simulink model "lptmr_complex_time_counter_s32k11x"  (Simulink 9.0)
settings: Solver=FixedStepDiscrete  StartTime=0.0  StopTime=10.0  FixedStep=0.1  RelTol=1e-3
InitFcn:
  | mbd_s32k_consistency_checks(bdroot(gcs));
undefined symbols (not defined in the file): LQFP, thumb
libraries: mbd_s32k1xx_ec_toolbox x12, simulink x1
Description:
  | This model demonstrates the "Low Power Timer" functionality by setting the peripheral to work in Time counter mode and using most of the LPTMR blocks.
  | 
  | Validation: When the processor boots up, it configures the LPTMR timer to Time Counter mode at an initial time period  of 1 sec and also enables the ISR. At every LPTMR
  |  interrup callback the model gets the compare value and toggles it between 50 or 950 msecs, so the RGB led will lightd up 50 msecs green at every second. On every step
  | function, the model gets the counter value and compares it to 55k Ticks and and the RGB led will lights up red if the counter value is higher than 50k Ticks. The counter can
  | be stopped if the SW3 switch is pressed and can be started if the SW2 switch is pressed.
settings Model: Creator=NXP MBDT Team  LastModifiedBy=nxf35172
settings DataIOCC: ExternalInput=off  InitialState=off  SaveFormat=Dataset  SaveOutput=off  SignalLogging=off  SaveTime=off
settings OptimizationCC: DefaultParameterBehavior=Inlined  PassReuseOutputArgsAs=Individual arguments  LifeSpan=auto
settings DebuggingCC: UnderspecifiedInitializationDetection=Simplified  MergeDetectMultiDrivingBlocksExec=error  InheritedTsInSrcMsg=none  SingleTaskRateTransMsg=error  ParameterTunabilityLossMsg=error  UnconnectedInputMsg=error  UnconnectedOutputMsg=error  UnconnectedLineMsg=error  UnknownTsInhSupMsg=error  SFUnexpectedBacktrackingDiag=error  SFNoUnconditionalDefaultTransitionDiag=error  SFExecutionAtInitializationDiag=warning
settings HardwareCC: ProdLargestAtomicInteger=Long  ProdLargestAtomicFloat=Double  ProdIntDivRoundTo=Zero  ProdEndianess=LittleEndian  ProdHWDeviceType=ARM Compatible->ARM Cortex
settings ModelReferenceCC: PropagateSignalLabelsOutOfModel=on
settings SFSimCC: MATLABDynamicMemAlloc=off
settings RTWCC: SystemTargetFile=mbd_s32k.tlc  MakeCommand=mbd_s32k_make_rtw COPY_MDLREF_INCLUDES=0  TemplateMakefile=mbd_s32k.tmf  Description=Model Based Design Toolbox S32K14x Code Generation Target  GenerateReport=on  IncludeHyperlinkInReport=on  LaunchReport=on  GenerateTraceInfo=on  GenerateTraceReport=on  GenerateTraceReportSl=on  GenerateTraceReportSf=on  GenerateTraceReportEml=on
settings CodeAppCC: ForceParamTrailComments=on  IgnoreCustomStorageClasses=off  OperatorAnnotations=on  SimulinkDataObjDesc=on  SFDataObjDesc=on  InsertBlockDesc=on  StateflowObjectComments=off
settings STFCustomTargetCC: TargetLangStandard=C99 (ISO)  MultiwordLength=256  CombineOutputUpdateFcns=on  ERTCustomFileBanners=on  SupportContinuousTime=off  SupportNonInlinedSFcns=off  RemoveResetFunc=on  MATLABClassNameForMDSCustomization=Simulink.SoftwareTarget.ERTCustomization  GRTInterface=off  SystemTargetFile=mbd_s32k.tlc
settings ERTTargetCC: TargetLangStandard=C99 (ISO)  ParMdlRefBuildCompliant=off  CompOptLevelCompliant=off  ConcurrentExecutionCompliant=off  ModelStepFunctionPrototypeControlCompliant=off  CPPClassGenCompliant=off  UseToolchainInfoCompliant=off  InlinedParameterPlacement=NonHierarchical  ERTSrcFileBannerTemplate=mbd_ert_code_template.cgt  ERTHdrFileBannerTemplate=mbd_ert_code_template.cgt  ERTDataSrcFileTemplate=mbd_ert_code_template.cgt  ERTDataHdrFileTemplate=mbd_ert_code_template.cgt  ERTCustomFileTemplate=example_file_process.tlc
settings ConfigComp: CovMetricSettings=dwe  CovHtmlReporting=off  CovSaveCumulativeToWorkspaceVar=off  CovSaveSingleToWorkspaceVar=off  CovExternalEMLEnable=on

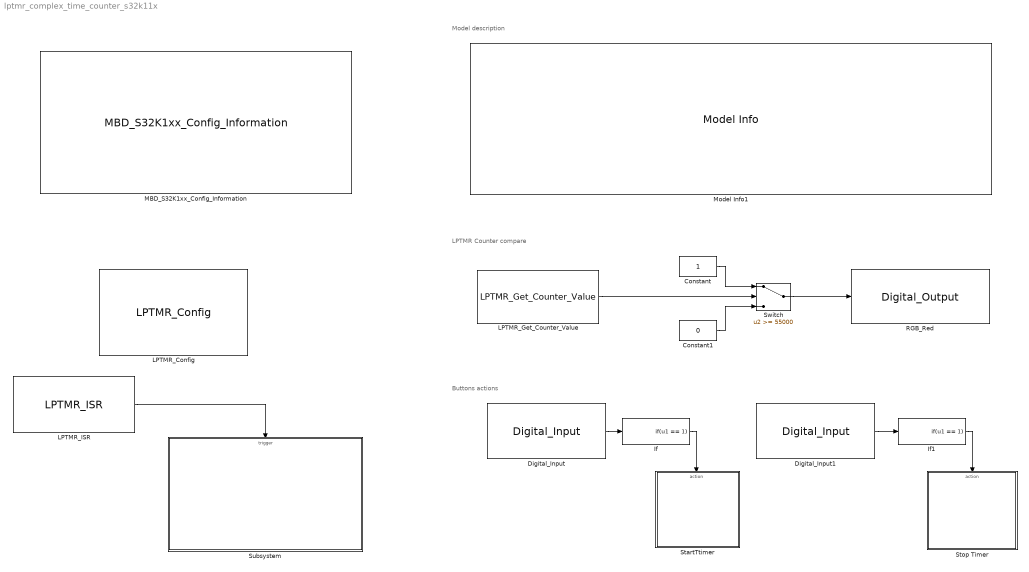
== system lptmr_complex_time_counter_s32k11x ==
  note: Buttons actions
  note: Model description
  note: LPTMR Counter compare
  Constant : Constant  OutDataTypeStr=boolean
  Constant1 : Constant  Value=0  OutDataTypeStr=boolean
  Digital_Input : mbd_s32k1xx_ec_toolbox/GPIO Blocks/Digital_Input  gpio_pin=PTD3: [PTD3 | Port D I/O]  pull_resistor=None  passive_filter=off
  Digital_Input1 : mbd_s32k1xx_ec_toolbox/GPIO Blocks/Digital_Input  gpio_pin=PTD5: [PTD5 | Port D I/O]  pull_resistor=None  passive_filter=off
  If : If  IfExpression=u1 == 1  ShowElse=off
  If1 : If  IfExpression=u1 == 1  ShowElse=off
  LPTMR_Config : mbd_s32k1xx_ec_toolbox/Core and System Blocks/LPTMR Blocks/LPTMR_Config  work_mode=Time Counter mode  compare_value=1000000  compare_value_units=Microseconds  pin_select=Count pulses from pin alternative 2  pin_polarity=Count pulse on rising edge  pin_trgmux_source=Trigger function is disabled  pin_gpio=PTE11: [LPTMR0_ALT1 | Low Power Timer Input Channel]  show_adv_opts=on  input_clock=SIRC DIV2 clock  prescaler=Timer mode: prescaler 2, Glitch filter mode: invalid  bypass_prescaler=off  free_run=off  start_counter=on  enable_isr=on
  LPTMR_Get_Counter_Value : mbd_s32k1xx_ec_toolbox/Core and System Blocks/LPTMR Blocks/LPTMR_Get_Counter_Value
  LPTMR_ISR : mbd_s32k1xx_ec_toolbox/Core and System Blocks/LPTMR Blocks/LPTMR_ISR
  MBD_S32K1xx_Config_Information : mbd_s32k1xx_ec_toolbox/MBD_S32K1xx_Config_Information  mbdt_ver=0  disp_str=|  config_params=[]  mcu_target_name=S32K116  mcu_target_package=48-LQFP  mcu_target_sram_size=17KB  mcu_system_clock_freq=40  mcu_xtal_freq=External 40  mcu_steptick_timer=LPIT Channel 0  mcu_steptick_prio=3  ds_import_enable=on  target_compiler=GCC  target_memory=FLASH  gcc_target_compile_opts=-mcpu=cortex-m0plus -mthumb -O1 -g -gstrict-dwarf  gcc_target_assemble_opts=-mcpu=cortex-m0plus -mthumb -g  gcc_target_link_opts=-mcpu=cortex-m0plus -mthumb  gcc_target_default_lcf=on  gcc_target_user_lcf=S32K116_17_flash.ld  ghs_target_compile_opts=-mcpu=cortexm0plus -mthumb -fsoft -Ogeneral -Wundef -Wimplicit-int -Wshadow -Wtrigraphs --no_commons --gnu_asm -gnu99 -gdwarf-2 -G  ghs_target_assemble_opts=-mcpu=cortexm0plus -mthumb -fsoft --gnu_asm  ghs_target_link_opts=-mcpu=cortexm0plus -mthumb -fsoft  ghs_target_default_lcf=on  ghs_target_user_lcf=S32K116_17_flash.ld  iar_target_compile_opts=--thumb -Ol -e --debug --dlib_config normal  iar_target_assemble_opts=--thumb  iar_target_link_opts=--no_exceptions --vfe --inline  iar_target_default_lcf=on  iar_target_user_lcf=S32K116_17_flash.icf  pil_download_enable=off  rbl_download_enable=on  rbl_start_delay=5000  rbl_download_interface=OpenSDA  rbl_restart_request=off  rbl_com_port=Custom  rbl_com_port_custom=COM1  pil_download_rate=57600  pil_opensda_drive=Custom  pil_opensda_drive_custom=D  pil_uart_instance=0  pil_uart_rx=PTA2: [LPUART0_RX | Receive]  pil_uart_tx=PTA3: [LPUART0_TX | Transmit]  FTM_PWM_PcrCheckEnDis=on  FTM_Input_Edge_Inputs_PcrCheckEnDis=on  FTM_Dual_Edge_Inputs_PcrCheckEnDis=on  FTM_Quadrature_Inputs_PcrCheckEnDis=on  FTM_Hall_Sensor_Inputs_PcrCheckEnDis=on  LPTMR_PcrCheckEnDis=on  PIT_PcrCheckEnDis=on  RTC_PcrCheckEnDis=on  FlexCAN_PcrCheckEnDis=on  LIN_PcrCheckEnDis=on  FlexIO_PcrCheckEnDis=on  LPI2C_PcrCheckEnDis=on  LPSPI_PcrCheckEnDis=on  LPUART_PcrCheckEnDis=on  CMP_PcrCheckEnDis=on  GPIO_OutputPcrCheckEnDis=on  GPIO_InputPcrCheckEnDis=on  SBC_PcrCheckEnDis=on  AMMCLIB_PcrCheckEnDis=on  FM_PcrCheckEnDis=on  Profile_PcrCheckEnDis=on  ConfigParams_PcrCheckEnDis=on  ModelRef_PcrCheckEnDis=on  PDB0_PcrCheckEnDis=on  CSEc_PcrCheckEnDis=on  eDMA_PcrCheckEnDis=on  ADC_PcrCheckEnDis=on  WDOG_PcrCheckEnDis=on
      | Target : S32K144-64KB_SRAM
      | Package : 100-pin
      | System clock : 80 MHz
      | XTAL clock : External 8 MHz
      | Compiler : IAR
      | Target Type : FLASH
      | Download Code after build : off
      | Step Tick Interrupt Priority : 15
  Model Info1 : simulink/Model-Wide Utilities/Model Info  Frame=off  DisplayStringWithTags=|  HorizontalTextAlignment=Left  LeftAlignmentValue=0.02
      | Model Name: %<ModelName>
      | 
      | Description: %<Description>
  RGB_Red : mbd_s32k1xx_ec_toolbox/GPIO Blocks/Digital_Output  gpio_pin=PTD16: [PTD16 | Port D I/O]  init_val=Low  drive_strength=Low
  StartTtimer : Subsystem
      settings: RTWSystemCode=Inline
  Stop Timer : Subsystem
      settings: RTWSystemCode=Inline
  Subsystem : Subsystem
  Switch : Switch  Threshold=55000
  wires:
  Digital_Input1/1 -> If1/1
  If1/1 -> Stop Timer/Action
  If/1 -> StartTtimer/Action
  LPTMR_Get_Counter_Value/1 -> Switch/2
  Digital_Input/1 -> If/1
  Constant/1 -> Switch/1
  Switch/1 -> RGB_Red/1
  Constant1/1 -> Switch/3
  LPTMR_ISR/1 -> Subsystem/Trigger

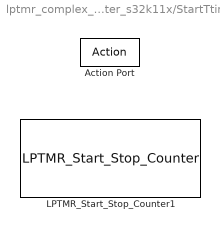
== system lptmr_complex_time_counter_s32k11x/StartTtimer ==
  Action Port : ActionPort
  LPTMR_Start_Stop_Counter1 : mbd_s32k1xx_ec_toolbox/Core and System Blocks/LPTMR Blocks/LPTMR_Start_Stop_Counter  set_action=Start

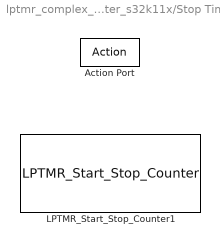
== system lptmr_complex_time_counter_s32k11x/Stop Timer ==
  Action Port : ActionPort
  LPTMR_Start_Stop_Counter1 : mbd_s32k1xx_ec_toolbox/Core and System Blocks/LPTMR Blocks/LPTMR_Start_Stop_Counter  set_action=Stop

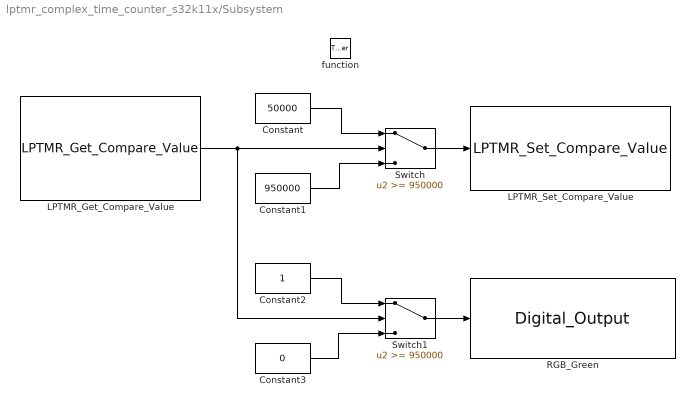
== system lptmr_complex_time_counter_s32k11x/Subsystem ==
  function : TriggerPort  TriggerType=function-call  VariantControl=Variant
  Constant : Constant  Value=50000  OutDataTypeStr=uint32
  Constant1 : Constant  Value=950000  OutDataTypeStr=uint32
  Constant2 : Constant  OutDataTypeStr=boolean
  Constant3 : Constant  Value=0  OutDataTypeStr=boolean
  LPTMR_Get_Compare_Value : mbd_s32k1xx_ec_toolbox/Core and System Blocks/LPTMR Blocks/LPTMR_Get_Compare_Value  Priority=1  compare_value_units=Microseconds
  LPTMR_Set_Compare_Value : mbd_s32k1xx_ec_toolbox/Core and System Blocks/LPTMR Blocks/LPTMR_Set_Compare_Value  Priority=9  compare_value_units=Microseconds
  RGB_Green : mbd_s32k1xx_ec_toolbox/GPIO Blocks/Digital_Output  Priority=3  gpio_pin=PTD15: [PTD15 | Port D I/O]  init_val=Low  drive_strength=Low
  Switch : Switch  Priority=5  Threshold=950000
  Switch1 : Switch  Threshold=950000
  wires:
  Switch/1 -> LPTMR_Set_Compare_Value/1
  Constant/1 -> Switch/1
  Constant1/1 -> Switch/3
  LPTMR_Get_Compare_Value/1 -> Switch1/2, Switch/2
  Switch1/1 -> RGB_Green/1
  Constant2/1 -> Switch1/1
  Constant3/1 -> Switch1/3
